simulink model "f6_Central_reservior_demo"  (R2019b)
settings: Solver=VariableStepAuto  StartTime=0.0  StopTime=3  RelTol=1e-3
undefined symbols (not defined in the file): Ion, Lithium
libraries: powerlib x86, powerlib_meascontrol x37, electricdrivelib x1
settings Model: SimulationMode=accelerator  Creator=HALUM  LastModifiedBy=MAHMUD
settings SolverCC: ZeroCrossAlgorithm=Adaptive  AlgebraicLoopSolver=LineSearch
settings DataIOCC: ReturnWorkspaceOutputs=off
settings DebuggingCC: MaskedZcDiagnostic=none  IgnoredZcDiagnostic=none  ArithmeticOperatorsInVariantConditions=warning
settings SFSimCC: SimUseLocalCustomCode=off  CustomCodeUndefinedFunction=UseInterfaceOnly
settings RTWCC: RTWUseLocalCustomCode=off

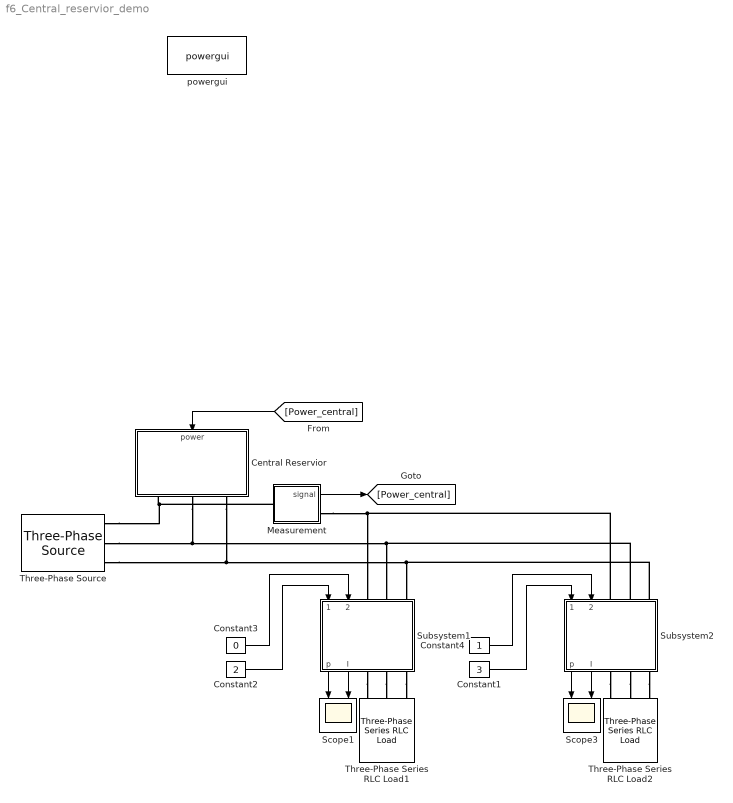
== system f6_Central_reservior_demo ==
  Central Reservior : Subsystem
  Constant1 : Constant  Value=3
  Constant2 : Constant  Value=2
  Constant3 : Constant  Value=0
  Constant4 : Constant
  Measurement : Subsystem
  Scope1 : Scope  NumInputPorts=2
  Scope3 : Scope  NumInputPorts=2
  Subsystem1 : Subsystem
  Subsystem2 : Subsystem
  Three-Phase Series RLC Load1 : powerlib/Elements/Three-Phase Series RLC Load  LConnTagsString=A|B|C  Configuration=Y (grounded)  NominalVoltage=220  Vabc=[1e3 1e3 1e3]  Vabcp=[1e3 1e3 1e3]  NominalFrequency=50  UnbalancedPower=off  ActivePower=200  InductivePower=0  CapacitivePower=0  Pabc=[10e3 9e3 11e3]  QLabc=[100 90 110]  QCabc=[100 90 110]  Pabcp=[10e3 9e3 11e3]  QLabcp=[100 90 110]  QCabcp=[100 90 110]  Measurements=None  LoadType=constant Z
      settings: SourceProductName=Simscape Electrical
  Three-Phase Series RLC Load2 : powerlib/Elements/Three-Phase Series RLC Load  LConnTagsString=A|B|C  Configuration=Y (grounded)  NominalVoltage=220  Vabc=[1e3 1e3 1e3]  Vabcp=[1e3 1e3 1e3]  NominalFrequency=50  UnbalancedPower=off  ActivePower=200  InductivePower=0  CapacitivePower=0  Pabc=[10e3 9e3 11e3]  QLabc=[100 90 110]  QCabc=[100 90 110]  Pabcp=[10e3 9e3 11e3]  QLabcp=[100 90 110]  QCabcp=[100 90 110]  Measurements=None  LoadType=constant Z
      settings: SourceProductName=Simscape Electrical
  Three-Phase Source : powerlib/Electrical Sources/Three-Phase Source  InternalConnection=Yg  VoltagePhases=off  Voltage=1986  PhaseAngle=0  Voltage_phases=[25e3 25e3 25e3]/sqrt(3)  PhaseAngles_phases=[0 -120 +120]  Frequency=50  NonIdealSource=off  SpecifyImpedance=off  Resistance=0.8929  Inductance=0  ShortCircuitLevel=100e6  BaseVoltage=1500  XRratio=7  BusType=swing  Pref=1e3  Qref=0  Prefabc=[10e3, 10e3, 10e3]  Qrefabc=[0, 0, 0]  Qmin=-inf  Qmax=inf
      settings: SourceProductName=Simscape Electrical
  powergui : powerlib/powergui  Priority=1  SimulationMode=Continuous  SampleTime=1e-2  frequency=60  Iterations=50  frequencyindice=50  Pbase=100e6  ErrMax=1e-4  UnitsV=kV  UnitsW=MW  buscounter=0  FunctionMessages=off  echomessages=off  EnableUseOfTLC=off  CurrentSourceSwitches=off  DisableSnubberDevices=off  DisableRonSwitches=off  DisableVfSwitches=off  DisplayEquations=off  AutomaticDiscreteSolvers=off  SolverType=Tustin/Backward Euler (TBE)  Interpol=off  ExternalGateDelay=off  methode=off  Ts=100  x0status=blocks  SPID=on  SwTol=0  HookPort=off  NonlinearTolerance=1e-4  nMaxIteration=100  ContinueOnMaxIteration=off  RestoreLinks=warning  ResistiveCurrentMeasurement=off  Frange=[0:2:500]  Ylog=off  Xlog=on  ShowGrid=off  save=off  variable=ZData  structure=0  ZoomFFT=off  StartTime=0.0  cycles=1  DisplayStyle=1  fundamental=60  FreqAxis=off  MaxFrequency=1000  frequencyindicesteady=1  RmsSteady=1  display=off
      settings: SourceProductName=Simscape Electrical
  wires:
  [Power_central] -> Central Reservior/1(power)
  Subsystem1/1(p) -> Scope1/1
  Subsystem1/2(I) -> Scope1/2
  Constant3/1 -> Subsystem1/2(start time)
  Constant2/1 -> Subsystem1/1(stop time)
  Measurement/1("signal ") -> [Power_central]
  Constant1/1 -> Subsystem2/1(stop time)
  Constant4/1 -> Subsystem2/2(start time)
  Subsystem2/2(I) -> Scope3/2
  Subsystem2/1(p) -> Scope3/1
  connections:
  Subsystem1/RConn3 -- Three-Phase Series RLC Load1/LConn3
  Subsystem1/RConn2 -- Three-Phase Series RLC Load1/LConn2
  Subsystem1/RConn1 -- Three-Phase Series RLC Load1/LConn1
  Central Reservior/RConn3 -- Three-Phase Source/RConn3 -- Subsystem2/LConn3 -- Subsystem1/LConn3
  Central Reservior/RConn2 -- Three-Phase Source/RConn2 -- Subsystem2/LConn2 -- Subsystem1/LConn2
  Measurement/RConn1 -- Subsystem2/LConn1 -- Subsystem1/LConn1
  Measurement/LConn1 -- Three-Phase Source/RConn1 -- Central Reservior/RConn1
  Subsystem2/RConn1 -- Three-Phase Series RLC Load2/LConn1
  Subsystem2/RConn2 -- Three-Phase Series RLC Load2/LConn2
  Subsystem2/RConn3 -- Three-Phase Series RLC Load2/LConn3

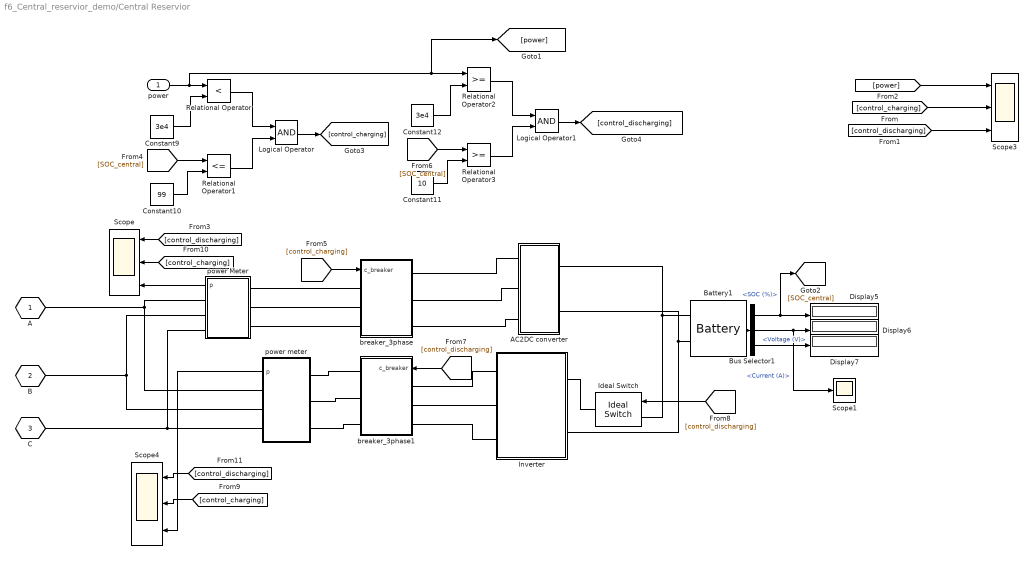
== system f6_Central_reservior_demo/Central Reservior ==
  power : Inport
  AC2DC converter : Subsystem
  Battery1 : electricdrivelib/Extra Sources/Battery  BatType=Lithium-Ion  ShowTempParam=off  ThermalPreset=no  ShowAgeParam=off  NomV=1000  NomQ=1000  SOC=80  Batt_Tr=0.1  PresetModel=on  MaxQ=1000  MinV=750  FullV=1163.9871  Dis_rate=434.7826  R=0.01  Normal_OP=904.3478  expZone="[1080.3859      49.130435]"  current=[6.5 13 32.5]  Units=Time  Tci=20  NomT=20  T2=-30  MaxQ2=4.8  FullV2=7.1  Normal_OP2=5.655  expZone2="[6.58           1]"  Rca=0.6  ti=2000  Dp=0  Neq0=0  Tsim=1e6  Ta1=25  Qeol=5.4*0.9  Reol=0.013333*1.2  Char_age=[2.3478, 3]  Dis_age=[2.3478, 10]  N1=1500  N2=10500  N3=1000  N4=1400  Ta2=45  N5=950
  Bus Selector1 : BusSelector  OutputSignals=SOC (%),Current (A),Voltage (V)
  Constant10 : Constant  Value=99
  Constant11 : Constant  Value=10
  Constant12 : Constant  Value=3e4
  Constant9 : Constant  Value=3e4
  Display5 : Display
  Display6 : Display
  Display7 : Display
  Ideal Switch : powerlib/Power Electronics/Ideal Switch  Ron=0.001  Lon=0  IC=0  Rs=1e5  Cs=inf  Measurements=off
      settings: SourceProductName=Simscape Electrical
  Inverter : Subsystem
  Logical Operator : Logic  AllPortsSameDT=off  OutDataTypeStr=boolean
  Logical Operator1 : Logic  AllPortsSameDT=off  OutDataTypeStr=boolean
  Relational Operator : RelationalOperator  Operator=<  OutDataTypeStr=boolean  ZeroCross=off  RndMeth=Simplest
  Relational Operator1 : RelationalOperator  Operator=<=  OutDataTypeStr=boolean  RndMeth=Simplest
  Relational Operator2 : RelationalOperator  OutDataTypeStr=boolean  ZeroCross=off  RndMeth=Simplest
  Relational Operator3 : RelationalOperator  OutDataTypeStr=boolean  RndMeth=Simplest
  Scope : Scope  NumInputPorts=3
  Scope1 : Scope
  Scope3 : Scope  NumInputPorts=3
  Scope4 : Scope  NumInputPorts=3
  breaker_3phase : Subsystem
  breaker_3phase1 : Subsystem
  power Meter : Subsystem
  power meter : Subsystem
  A : PMIOPort  Tag=PMCPort  Side=Right
  B : PMIOPort  Tag=PMCPort  Port=2  Side=Right
  C : PMIOPort  Tag=PMCPort  Port=3  Side=Right
  wires:
  power/1 -> [power], Relational Operator2/1, Relational Operator/1
  Bus Selector1/2 -> Scope1/1, Display6/1  "<Current (A)>"
  Bus Selector1/3 -> Display7/1  "<Voltage (V)>"
  Battery1/1 -> Bus Selector1/1
  [SOC_central] -> Relational Operator3/1
  Bus Selector1/1 -> [SOC_central], Display5/1  "<SOC (%)>"
  Constant9/1 -> Relational Operator/2
  Logical Operator/1 -> [control_charging]
  Constant10/1 -> Relational Operator1/2
  [SOC_central] -> Relational Operator1/1
  Logical Operator1/1 -> [control_discharging]
  Relational Operator2/1 -> Logical Operator1/1
  Relational Operator1/1 -> Logical Operator/2
  Relational Operator3/1 -> Logical Operator1/2
  Constant11/1 -> Relational Operator3/2
  Constant12/1 -> Relational Operator2/2
  [control_charging] -> breaker_3phase/1(c_breaker)
  [control_discharging] -> Ideal Switch/1
  [control_discharging] -> breaker_3phase1/1(c_breaker)
  Relational Operator/1 -> Logical Operator/1
  [control_discharging] -> Scope3/3
  [control_charging] -> Scope3/2
  [power] -> Scope3/1
  power Meter/1(p) -> Scope/3
  [control_charging] -> Scope/2
  [control_discharging] -> Scope/1
  [control_discharging] -> Scope4/1
  [control_charging] -> Scope4/2
  power meter/1(p) -> Scope4/3
  connections:
  breaker_3phase/RConn3 -- AC2DC converter/LConn3
  Battery1/LConn1 -- Ideal Switch/LConn1 -- AC2DC converter/RConn1
  breaker_3phase/RConn2 -- AC2DC converter/LConn2
  Battery1/LConn2 -- Inverter/LConn2 -- AC2DC converter/RConn2
  breaker_3phase/RConn1 -- AC2DC converter/LConn1
  Ideal Switch/RConn1 -- Inverter/LConn1
  breaker_3phase1/LConn1 -- Inverter/RConn1
  breaker_3phase1/LConn3 -- Inverter/RConn3
  breaker_3phase1/LConn2 -- Inverter/RConn2
  power meter/LConn2 -- breaker_3phase1/RConn2
  power meter/LConn1 -- breaker_3phase1/RConn1
  power meter/LConn3 -- breaker_3phase1/RConn3
  power Meter/LConn3 -- breaker_3phase/LConn3
  power Meter/LConn2 -- breaker_3phase/LConn2
  power Meter/LConn1 -- breaker_3phase/LConn1
  power Meter/RConn1 -- power meter/RConn1 -- A/RConn1
  power Meter/RConn2 -- power meter/RConn2 -- B/RConn1
  power Meter/RConn3 -- power meter/RConn3 -- C/RConn1

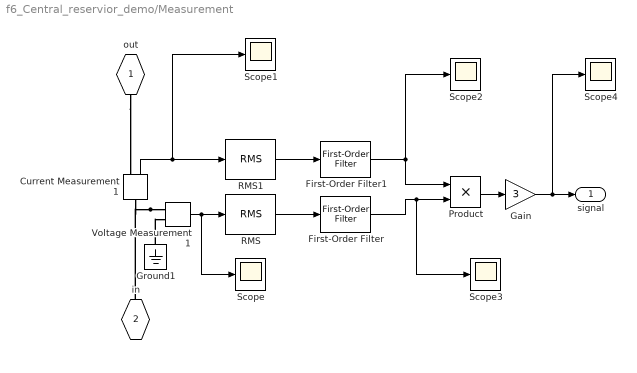
== system f6_Central_reservior_demo/Measurement ==
  Current Measurement1 : powerlib/Measurements/Current Measurement  PhasorSimulation=off  OutputType=Complex  PSBequivalent=0
      settings: SourceProductName=Simscape Electrical
  First-Order Filter : powerlib_meascontrol/Filters/First-Order Filter  FilterType=Lowpass  Tc=100e-3  Ts=0  Initialize=off  Vac_Init=[0, 0, 50]  Vdc_Init=0  PlotResponse=off  FreqRange="[0,  200,  1]"
      settings: SourceProductName=Simscape Electrical
  First-Order Filter1 : powerlib_meascontrol/Filters/First-Order Filter  FilterType=Lowpass  Tc=100e-3  Ts=0  Initialize=off  Vac_Init=[0, 0, 50]  Vdc_Init=0  PlotResponse=off  FreqRange="[0,  200,  1]"
      settings: SourceProductName=Simscape Electrical
  Gain : Gain  Gain=3
  Ground1 : powerlib/Elements/Ground  LConnTagsString=a
      settings: SourceProductName=Simscape Electrical
  Product : Product
  RMS : powerlib_meascontrol/Measurements/RMS  TrueRMS=on  Freq=50  RMSInit=210  Ts=0.001
      settings: SourceProductName=Simscape Electrical
  RMS1 : powerlib_meascontrol/Measurements/RMS  TrueRMS=on  Freq=50  RMSInit=210  Ts=0.001
      settings: SourceProductName=Simscape Electrical
  Scope{,1..4} (5 alike) : Scope
  Voltage Measurement1 : powerlib/Measurements/Voltage Measurement  PhasorSimulation=off  OutputType=Complex  PSBequivalent=0
      settings: SourceProductName=Simscape Electrical
  "out " : PMIOPort  Tag=PMCPort  Side=Right
  in : PMIOPort  Tag=PMCPort  Port=2  Side=Left
  "signal " : Outport
  wires:
  Product/1 -> Gain/1
  First-Order Filter/1 -> Product/2, Scope3/1
  First-Order Filter1/1 -> Scope2/1, Product/1
  Voltage Measurement1/1 -> RMS/1, Scope/1
  RMS1/1 -> First-Order Filter1/1
  RMS/1 -> First-Order Filter/1
  Gain/1 -> Scope4/1, "signal "/1
  Current Measurement1/1 -> RMS1/1, Scope1/1
  connections:
  "out "/RConn1 -- Current Measurement1/RConn1
  Voltage Measurement1/LConn1 -- in/RConn1 -- Current Measurement1/LConn1
  Ground1/LConn1 -- Voltage Measurement1/LConn2

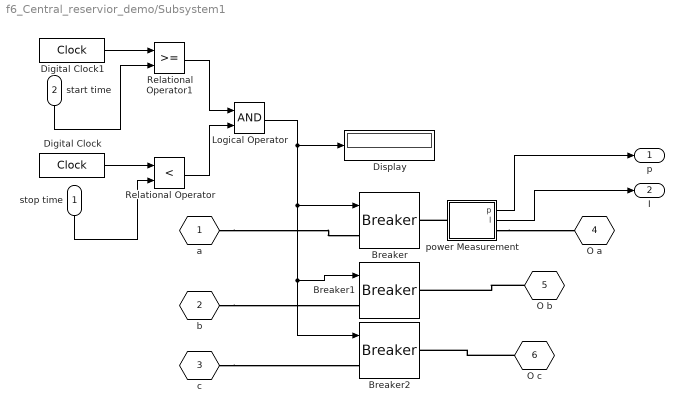
== system f6_Central_reservior_demo/Subsystem1 ==
  stop time : Inport
  start time : Inport  Port=2
  Breaker : powerlib/Elements/Breaker  InitialState=0  SwitchingTimes="[1/60  5/60]"  External=on  BreakerResistance=0.01  SnubberResistance=1e6  SnubberCapacitance=inf  Measurements=None  MoreParameters=on  NoBreakLoop=off
      settings: SourceProductName=Simscape Electrical
  Breaker1 : powerlib/Elements/Breaker  InitialState=0  SwitchingTimes="[1/60  5/60]"  External=on  BreakerResistance=0.01  SnubberResistance=1e6  SnubberCapacitance=inf  Measurements=None  MoreParameters=on  NoBreakLoop=off
      settings: SourceProductName=Simscape Electrical
  Breaker2 : powerlib/Elements/Breaker  InitialState=0  SwitchingTimes="[1/60  5/60]"  External=on  BreakerResistance=0.01  SnubberResistance=1e6  SnubberCapacitance=inf  Measurements=None  MoreParameters=on  NoBreakLoop=off
      settings: SourceProductName=Simscape Electrical
  Digital Clock : DigitalClock
  Digital Clock1 : DigitalClock
  Display : Display
  Logical Operator : Logic  AllPortsSameDT=off  OutDataTypeStr=boolean
  Relational Operator : RelationalOperator  Operator=<  OutDataTypeStr=boolean  RndMeth=Simplest
  Relational Operator1 : RelationalOperator  OutDataTypeStr=boolean  RndMeth=Simplest
  power Measurement : Subsystem
  a : PMIOPort  Tag=PMCPort  Side=Left
  b : PMIOPort  Tag=PMCPort  Port=2  Side=Left
  c : PMIOPort  Tag=PMCPort  Port=3  Side=Left
  "O a " : PMIOPort  Tag=PMCPort  Port=4  Side=Right
  O b : PMIOPort  Tag=PMCPort  Port=5  Side=Right
  O c : PMIOPort  Tag=PMCPort  Port=6  Side=Right
  p : Outport
  I : Outport  Port=2
  wires:
  power Measurement/1(p) -> p/1
  power Measurement/2(I) -> I/1
  Logical Operator/1 -> Breaker/1, Breaker2/1, Breaker1/1, Display/1
  Digital Clock/1 -> Relational Operator/1
  stop time/1 -> Relational Operator/2
  Digital Clock1/1 -> Relational Operator1/1
  start time/1 -> Relational Operator1/2
  Relational Operator1/1 -> Logical Operator/1
  Relational Operator/1 -> Logical Operator/2
  connections:
  power Measurement/LConn1 -- Breaker/RConn1
  power Measurement/RConn1 -- "O a "/RConn1
  O c/RConn1 -- Breaker2/RConn1
  b/RConn1 -- Breaker1/LConn1
  O b/RConn1 -- Breaker1/RConn1
  c/RConn1 -- Breaker2/LConn1
  a/RConn1 -- Breaker/LConn1

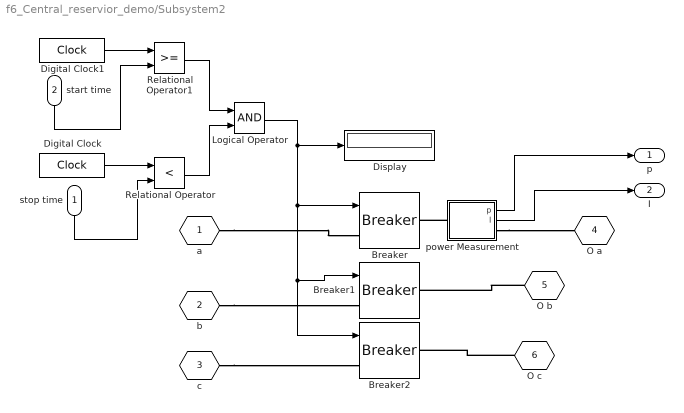
== system f6_Central_reservior_demo/Subsystem2 ==
  stop time : Inport
  start time : Inport  Port=2
  Breaker : powerlib/Elements/Breaker  InitialState=0  SwitchingTimes="[1/60  5/60]"  External=on  BreakerResistance=0.01  SnubberResistance=1e6  SnubberCapacitance=inf  Measurements=None  MoreParameters=on  NoBreakLoop=off
      settings: SourceProductName=Simscape Electrical
  Breaker1 : powerlib/Elements/Breaker  InitialState=0  SwitchingTimes="[1/60  5/60]"  External=on  BreakerResistance=0.01  SnubberResistance=1e6  SnubberCapacitance=inf  Measurements=None  MoreParameters=on  NoBreakLoop=off
      settings: SourceProductName=Simscape Electrical
  Breaker2 : powerlib/Elements/Breaker  InitialState=0  SwitchingTimes="[1/60  5/60]"  External=on  BreakerResistance=0.01  SnubberResistance=1e6  SnubberCapacitance=inf  Measurements=None  MoreParameters=on  NoBreakLoop=off
      settings: SourceProductName=Simscape Electrical
  Digital Clock : DigitalClock
  Digital Clock1 : DigitalClock
  Display : Display
  Logical Operator : Logic  AllPortsSameDT=off  OutDataTypeStr=boolean
  Relational Operator : RelationalOperator  Operator=<  OutDataTypeStr=boolean  RndMeth=Simplest
  Relational Operator1 : RelationalOperator  OutDataTypeStr=boolean  RndMeth=Simplest
  power Measurement : Subsystem
  a : PMIOPort  Tag=PMCPort  Side=Left
  b : PMIOPort  Tag=PMCPort  Port=2  Side=Left
  c : PMIOPort  Tag=PMCPort  Port=3  Side=Left
  "O a " : PMIOPort  Tag=PMCPort  Port=4  Side=Right
  O b : PMIOPort  Tag=PMCPort  Port=5  Side=Right
  O c : PMIOPort  Tag=PMCPort  Port=6  Side=Right
  p : Outport
  I : Outport  Port=2
  wires:
  Relational Operator/1 -> Logical Operator/2
  Relational Operator1/1 -> Logical Operator/1
  start time/1 -> Relational Operator1/2
  Digital Clock1/1 -> Relational Operator1/1
  stop time/1 -> Relational Operator/2
  Digital Clock/1 -> Relational Operator/1
  Logical Operator/1 -> Display/1, Breaker1/1, Breaker2/1, Breaker/1
  power Measurement/2(I) -> I/1
  power Measurement/1(p) -> p/1
  connections:
  a/RConn1 -- Breaker/LConn1
  c/RConn1 -- Breaker2/LConn1
  O b/RConn1 -- Breaker1/RConn1
  b/RConn1 -- Breaker1/LConn1
  O c/RConn1 -- Breaker2/RConn1
  power Measurement/RConn1 -- "O a "/RConn1
  power Measurement/LConn1 -- Breaker/RConn1

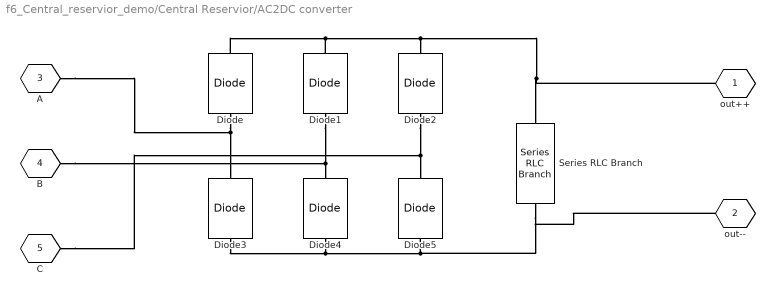
== system f6_Central_reservior_demo/Central Reservior/AC2DC converter ==
  Diode{,1..5} (6 alike) : powerlib/Power Electronics/Diode  Ron=0.001  Lon=0  Vf=0.8  IC=0  UseSnubber=0  Rs=500  Cs=250e-9  Measurements=off
      settings: SourceProductName=Simscape Electrical
  Series RLC Branch : powerlib/Elements/Series RLC Branch  LConnTagsString=__new0  RConnTagsString=__new0  BranchType=C  Resistance=1  Inductance=1e-3  SetiL0=off  InitialCurrent=0  Capacitance=220e-6  Setx0=off  InitialVoltage=0  Measurements=None
      settings: SourceProductName=Simscape Electrical
  out++ : PMIOPort  Tag=PMCPort  Side=Right
  out-- : PMIOPort  Tag=PMCPort  Port=2  Side=Right
  A : PMIOPort  Tag=PMCPort  Port=3  Side=Left
  B : PMIOPort  Tag=PMCPort  Port=4  Side=Left
  C : PMIOPort  Tag=PMCPort  Port=5  Side=Left
  connections:
  Diode/RConn1 -- Diode1/RConn1 -- out++/RConn1 -- Series RLC Branch/RConn1 -- Diode2/RConn1
  Diode3/LConn1 -- Diode4/LConn1 -- out--/RConn1 -- Series RLC Branch/LConn1 -- Diode5/LConn1
  Diode1/LConn1 -- B/RConn1 -- Diode4/RConn1
  Diode/LConn1 -- A/RConn1 -- Diode3/RConn1
  Diode2/LConn1 -- C/RConn1 -- Diode5/RConn1

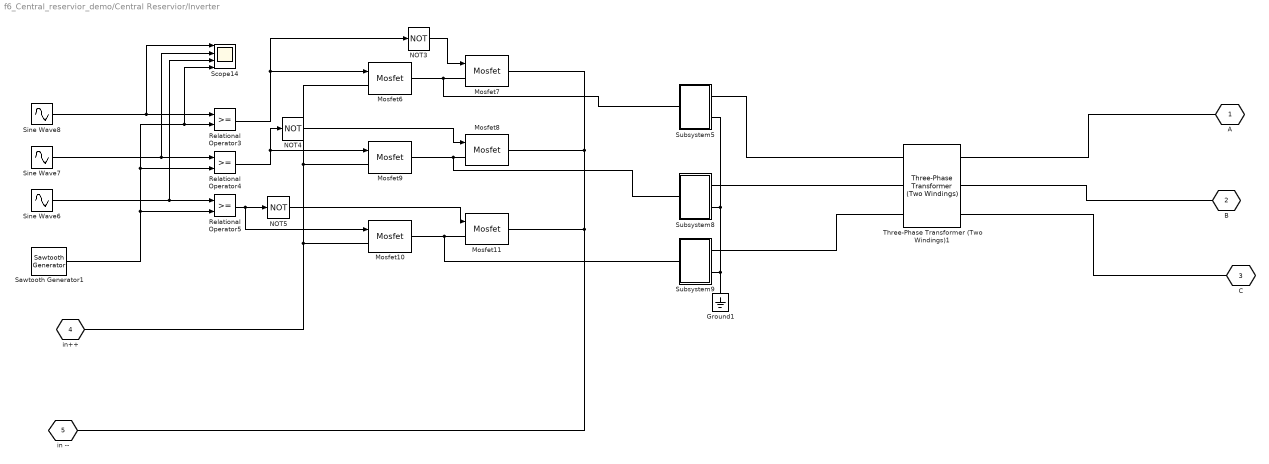
== system f6_Central_reservior_demo/Central Reservior/Inverter ==
  Ground1 : powerlib/Elements/Ground  LConnTagsString=a
      settings: SourceProductName=Simscape Electrical
  Mosfet{6..11} (6 alike) : powerlib/Power Electronics/Mosfet  Ron=0.1  Lon=0  Rd=0.01  Vfd=0  IC=0  Rs=1e5  Cs=inf  Measurements=off
      settings: SourceProductName=Simscape Electrical
  NOT3 : Logic  Operator=NOT  IconShape=distinctive  AllPortsSameDT=off  OutDataTypeStr=boolean
  NOT4 : Logic  Operator=NOT  IconShape=distinctive  AllPortsSameDT=off  OutDataTypeStr=boolean
  NOT5 : Logic  Operator=NOT  IconShape=distinctive  AllPortsSameDT=off  OutDataTypeStr=boolean
  Relational Operator3 : RelationalOperator  OutDataTypeStr=boolean  RndMeth=Simplest
  Relational Operator4 : RelationalOperator  OutDataTypeStr=boolean  RndMeth=Simplest
  Relational Operator5 : RelationalOperator  OutDataTypeStr=boolean  RndMeth=Simplest
  Sawtooth Generator1 : powerlib_meascontrol/Pulse & Signal Generators/Sawtooth Generator  Freq=1e3  Phase=180  Ts=0
      settings: SourceProductName=Simscape Electrical
  Scope14 : Scope  NumInputPorts=4
  Sine Wave6 : Sin  Frequency=2*pi*50  Phase=4*pi/3  SampleTime=0
  Sine Wave7 : Sin  Frequency=2*pi*50  Phase=2*pi/3  SampleTime=0
  Sine Wave8 : Sin  Frequency=2*pi*50  SampleTime=0
  Subsystem5 : Subsystem
  Subsystem8 : Subsystem
  Subsystem9 : Subsystem
  Three-Phase Transformer (Two Windings)1 : powerlib/Elements/Three-Phase Transformer (Two Windings)  Winding1Connection=Yg  Winding2Connection=Yg  CoreType=Three single-phase transformers  SetSaturation=off  Hysteresis=off  DataFile='hysteresis'  SetInitialFlux=off  Measurements=None  UNITS=pu  NominalPower=[ 100e3 , 50 ]  Winding1=[ 338 , 0.002 , 0.08 ]  Winding2=[ 1200 , 0.002 , 0.08 ]  Rm=500  Lm=500  L0=0.5  Saturation=[ 0,0 ; 0.0024,1.2 ; 1.0,1.52 ]  InitialFluxes=[ 0.8 , -0.8 , 0.7 ]  BreakLoop=off  DiscreteSolver=Trapezoidal iterative  DataType=off  TransfoNumber=1
      settings: SourceProductName=Simscape Electrical
  A : PMIOPort  Tag=PMCPort  Side=Right
  B : PMIOPort  Tag=PMCPort  Port=2  Side=Right
  C : PMIOPort  Tag=PMCPort  Port=3  Side=Right
  in++ : PMIOPort  Tag=PMCPort  Port=4  Side=Left
  in -- : PMIOPort  Tag=PMCPort  Port=5  Side=Left
  wires:
  Relational Operator3/1 -> Mosfet6/1, NOT3/1
  Relational Operator5/1 -> NOT5/1, Mosfet10/1
  NOT3/1 -> Mosfet7/1
  Sine Wave8/1 -> Scope14/1, Relational Operator3/1
  Sawtooth Generator1/1 -> Relational Operator5/2, Relational Operator4/2, Scope14/4, Relational Operator3/2
  NOT4/1 -> Mosfet8/1
  Relational Operator4/1 -> NOT4/1, Mosfet9/1
  Sine Wave7/1 -> Scope14/2, Relational Operator4/1
  Sine Wave6/1 -> Scope14/3, Relational Operator5/1
  NOT5/1 -> Mosfet11/1
  connections:
  Subsystem5/RConn2 -- Subsystem8/RConn2 -- Ground1/LConn1 -- Subsystem9/RConn2
  Mosfet11/RConn1 -- in --/RConn1 -- Mosfet8/RConn1 -- Mosfet7/RConn1
  Subsystem5/LConn1 -- Mosfet7/LConn1 -- Mosfet6/RConn1
  Subsystem5/RConn1 -- Three-Phase Transformer (Two Windings)1/LConn1
  Subsystem9/LConn1 -- Mosfet10/RConn1 -- Mosfet11/LConn1
  Three-Phase Transformer (Two Windings)1/LConn2 -- Subsystem8/RConn1
  Subsystem8/LConn1 -- Mosfet8/LConn1 -- Mosfet9/RConn1
  Three-Phase Transformer (Two Windings)1/LConn3 -- Subsystem9/RConn1
  Mosfet6/LConn1 -- Mosfet9/LConn1 -- in++/RConn1 -- Mosfet10/LConn1
  Three-Phase Transformer (Two Windings)1/RConn1 -- A/RConn1
  Three-Phase Transformer (Two Windings)1/RConn2 -- B/RConn1
  Three-Phase Transformer (Two Windings)1/RConn3 -- C/RConn1

== system f6_Central_reservior_demo/Central Reservior/breaker_3phase ==
  c_breaker : Inport
  Breaker : powerlib/Elements/Breaker  InitialState=0  SwitchingTimes="[1/60  5/60]"  External=on  BreakerResistance=0.01  SnubberResistance=1e6  SnubberCapacitance=inf  Measurements=None  MoreParameters=on  NoBreakLoop=off
      settings: SourceProductName=Simscape Electrical
  Breaker1 : powerlib/Elements/Breaker  InitialState=0  SwitchingTimes="[1/60  5/60]"  External=on  BreakerResistance=0.01  SnubberResistance=1e6  SnubberCapacitance=inf  Measurements=None  MoreParameters=on  NoBreakLoop=off
      settings: SourceProductName=Simscape Electrical
  Breaker2 : powerlib/Elements/Breaker  InitialState=0  SwitchingTimes="[1/60  5/60]"  External=on  BreakerResistance=0.01  SnubberResistance=1e6  SnubberCapacitance=inf  Measurements=None  MoreParameters=on  NoBreakLoop=off
      settings: SourceProductName=Simscape Electrical
  a : PMIOPort  Tag=PMCPort  Side=Right
  A : PMIOPort  Tag=PMCPort  Port=2  Side=Left
  B : PMIOPort  Tag=PMCPort  Port=3  Side=Left
  C : PMIOPort  Tag=PMCPort  Port=4  Side=Left
  b : PMIOPort  Tag=PMCPort  Port=5  Side=Right
  c : PMIOPort  Tag=PMCPort  Port=6  Side=Right
  wires:
  c_breaker/1 -> Breaker2/1, Breaker1/1, Breaker/1
  connections:
  C/RConn1 -- Breaker2/LConn1
  b/RConn1 -- Breaker1/RConn1
  a/RConn1 -- Breaker/RConn1
  c/RConn1 -- Breaker2/RConn1
  A/RConn1 -- Breaker/LConn1
  B/RConn1 -- Breaker1/LConn1

== system f6_Central_reservior_demo/Central Reservior/breaker_3phase1 ==
  c_breaker : Inport
  Breaker : powerlib/Elements/Breaker  InitialState=0  SwitchingTimes="[1/60  5/60]"  External=on  BreakerResistance=0.01  SnubberResistance=1e6  SnubberCapacitance=inf  Measurements=None  MoreParameters=on  NoBreakLoop=off
      settings: SourceProductName=Simscape Electrical
  Breaker1 : powerlib/Elements/Breaker  InitialState=0  SwitchingTimes="[1/60  5/60]"  External=on  BreakerResistance=0.01  SnubberResistance=1e6  SnubberCapacitance=inf  Measurements=None  MoreParameters=on  NoBreakLoop=off
      settings: SourceProductName=Simscape Electrical
  Breaker2 : powerlib/Elements/Breaker  InitialState=0  SwitchingTimes="[1/60  5/60]"  External=on  BreakerResistance=0.01  SnubberResistance=1e6  SnubberCapacitance=inf  Measurements=None  MoreParameters=on  NoBreakLoop=off
      settings: SourceProductName=Simscape Electrical
  a : PMIOPort  Tag=PMCPort  Side=Right
  A : PMIOPort  Tag=PMCPort  Port=2  Side=Left
  B : PMIOPort  Tag=PMCPort  Port=3  Side=Left
  C : PMIOPort  Tag=PMCPort  Port=4  Side=Left
  b : PMIOPort  Tag=PMCPort  Port=5  Side=Right
  c : PMIOPort  Tag=PMCPort  Port=6  Side=Right
  wires:
  c_breaker/1 -> Breaker/1, Breaker1/1, Breaker2/1
  connections:
  B/RConn1 -- Breaker1/LConn1
  A/RConn1 -- Breaker/LConn1
  c/RConn1 -- Breaker2/RConn1
  a/RConn1 -- Breaker/RConn1
  b/RConn1 -- Breaker1/RConn1
  C/RConn1 -- Breaker2/LConn1

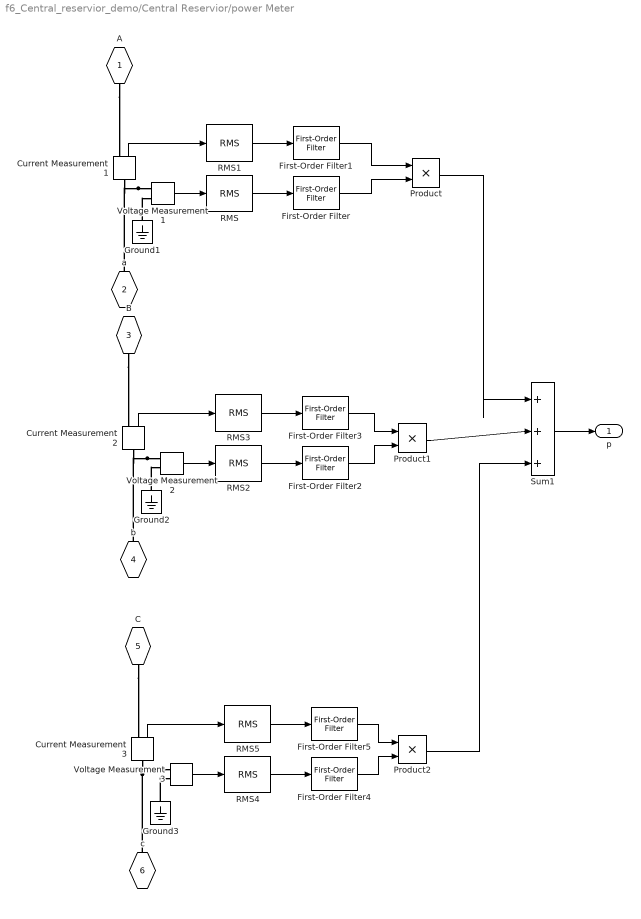
== system f6_Central_reservior_demo/Central Reservior/power Meter ==
  Current Measurement1 : powerlib/Measurements/Current Measurement  PhasorSimulation=off  OutputType=Complex  PSBequivalent=0
      settings: SourceProductName=Simscape Electrical
  Current Measurement2 : powerlib/Measurements/Current Measurement  PhasorSimulation=off  OutputType=Complex  PSBequivalent=0
      settings: SourceProductName=Simscape Electrical
  Current Measurement3 : powerlib/Measurements/Current Measurement  PhasorSimulation=off  OutputType=Complex  PSBequivalent=0
      settings: SourceProductName=Simscape Electrical
  First-Order Filter{,1..5} (6 alike) : powerlib_meascontrol/Filters/First-Order Filter  FilterType=Lowpass  Tc=100e-3  Ts=0  Initialize=off  Vac_Init=[0, 0, 50]  Vdc_Init=0  PlotResponse=off  FreqRange="[0,  200,  1]"
      settings: SourceProductName=Simscape Electrical
  Ground1 : powerlib/Elements/Ground  LConnTagsString=a
      settings: SourceProductName=Simscape Electrical
  Ground2 : powerlib/Elements/Ground  LConnTagsString=a
      settings: SourceProductName=Simscape Electrical
  Ground3 : powerlib/Elements/Ground  LConnTagsString=a
      settings: SourceProductName=Simscape Electrical
  Product : Product
  Product1 : Product
  Product2 : Product
  RMS{,1..5} (6 alike) : powerlib_meascontrol/Measurements/RMS  TrueRMS=on  Freq=50  RMSInit=210  Ts=0.001
      settings: SourceProductName=Simscape Electrical
  Sum1 : Sum  Inputs=|+++
  Voltage Measurement1 : powerlib/Measurements/Voltage Measurement  PhasorSimulation=off  OutputType=Complex  PSBequivalent=0
      settings: SourceProductName=Simscape Electrical
  Voltage Measurement2 : powerlib/Measurements/Voltage Measurement  PhasorSimulation=off  OutputType=Complex  PSBequivalent=0
      settings: SourceProductName=Simscape Electrical
  Voltage Measurement3 : powerlib/Measurements/Voltage Measurement  PhasorSimulation=off  OutputType=Complex  PSBequivalent=0
      settings: SourceProductName=Simscape Electrical
  "A " : PMIOPort  Tag=PMCPort  Side=Right
  a : PMIOPort  Tag=PMCPort  Port=2  Side=Left
  B : PMIOPort  Tag=PMCPort  Port=3  Side=Right
  b : PMIOPort  Tag=PMCPort  Port=4  Side=Left
  C : PMIOPort  Tag=PMCPort  Port=5  Side=Right
  c : PMIOPort  Tag=PMCPort  Port=6  Side=Left
  p : Outport
  wires:
  Product2/1 -> Sum1/3
  Product1/1 -> Sum1/2
  First-Order Filter4/1 -> Product2/2
  First-Order Filter5/1 -> Product2/1
  First-Order Filter2/1 -> Product1/2
  First-Order Filter3/1 -> Product1/1
  Voltage Measurement3/1 -> RMS4/1
  RMS5/1 -> First-Order Filter5/1
  RMS4/1 -> First-Order Filter4/1
  Current Measurement3/1 -> RMS5/1
  Current Measurement2/1 -> RMS3/1
  RMS2/1 -> First-Order Filter2/1
  RMS3/1 -> First-Order Filter3/1
  Voltage Measurement2/1 -> RMS2/1
  Product/1 -> Sum1/1
  First-Order Filter/1 -> Product/2
  First-Order Filter1/1 -> Product/1
  Voltage Measurement1/1 -> RMS/1
  RMS1/1 -> First-Order Filter1/1
  RMS/1 -> First-Order Filter/1
  Sum1/1 -> p/1
  Current Measurement1/1 -> RMS1/1
  connections:
  C/RConn1 -- Current Measurement3/RConn1
  Ground3/LConn1 -- Voltage Measurement3/LConn2
  Current Measurement3/LConn1 -- Voltage Measurement3/LConn1 -- c/RConn1
  Ground2/LConn1 -- Voltage Measurement2/LConn2
  B/RConn1 -- Current Measurement2/RConn1
  Voltage Measurement2/LConn1 -- Current Measurement2/LConn1 -- b/RConn1
  "A "/RConn1 -- Current Measurement1/RConn1
  Voltage Measurement1/LConn1 -- a/RConn1 -- Current Measurement1/LConn1
  Ground1/LConn1 -- Voltage Measurement1/LConn2

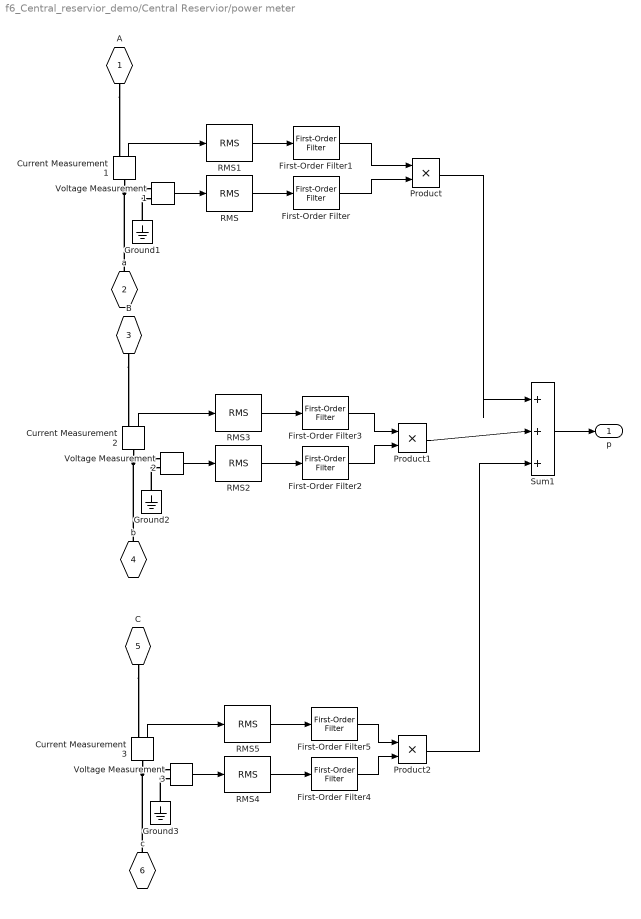
== system f6_Central_reservior_demo/Central Reservior/power meter ==
  Current Measurement1 : powerlib/Measurements/Current Measurement  PhasorSimulation=off  OutputType=Complex  PSBequivalent=0
      settings: SourceProductName=Simscape Electrical
  Current Measurement2 : powerlib/Measurements/Current Measurement  PhasorSimulation=off  OutputType=Complex  PSBequivalent=0
      settings: SourceProductName=Simscape Electrical
  Current Measurement3 : powerlib/Measurements/Current Measurement  PhasorSimulation=off  OutputType=Complex  PSBequivalent=0
      settings: SourceProductName=Simscape Electrical
  First-Order Filter{,1..5} (6 alike) : powerlib_meascontrol/Filters/First-Order Filter  FilterType=Lowpass  Tc=100e-3  Ts=0  Initialize=off  Vac_Init=[0, 0, 50]  Vdc_Init=0  PlotResponse=off  FreqRange="[0,  200,  1]"
      settings: SourceProductName=Simscape Electrical
  Ground1 : powerlib/Elements/Ground  LConnTagsString=a
      settings: SourceProductName=Simscape Electrical
  Ground2 : powerlib/Elements/Ground  LConnTagsString=a
      settings: SourceProductName=Simscape Electrical
  Ground3 : powerlib/Elements/Ground  LConnTagsString=a
      settings: SourceProductName=Simscape Electrical
  Product : Product
  Product1 : Product
  Product2 : Product
  RMS{,1..5} (6 alike) : powerlib_meascontrol/Measurements/RMS  TrueRMS=on  Freq=50  RMSInit=210  Ts=0.001
      settings: SourceProductName=Simscape Electrical
  Sum1 : Sum  Inputs=|+++
  Voltage Measurement1 : powerlib/Measurements/Voltage Measurement  PhasorSimulation=off  OutputType=Complex  PSBequivalent=0
      settings: SourceProductName=Simscape Electrical
  Voltage Measurement2 : powerlib/Measurements/Voltage Measurement  PhasorSimulation=off  OutputType=Complex  PSBequivalent=0
      settings: SourceProductName=Simscape Electrical
  Voltage Measurement3 : powerlib/Measurements/Voltage Measurement  PhasorSimulation=off  OutputType=Complex  PSBequivalent=0
      settings: SourceProductName=Simscape Electrical
  "A " : PMIOPort  Tag=PMCPort  Side=Right
  a : PMIOPort  Tag=PMCPort  Port=2  Side=Left
  B : PMIOPort  Tag=PMCPort  Port=3  Side=Right
  b : PMIOPort  Tag=PMCPort  Port=4  Side=Left
  C : PMIOPort  Tag=PMCPort  Port=5  Side=Right
  c : PMIOPort  Tag=PMCPort  Port=6  Side=Left
  p : Outport
  wires:
  Current Measurement1/1 -> RMS1/1
  Sum1/1 -> p/1
  RMS/1 -> First-Order Filter/1
  RMS1/1 -> First-Order Filter1/1
  Voltage Measurement1/1 -> RMS/1
  First-Order Filter1/1 -> Product/1
  First-Order Filter/1 -> Product/2
  Product/1 -> Sum1/1
  Voltage Measurement2/1 -> RMS2/1
  RMS3/1 -> First-Order Filter3/1
  RMS2/1 -> First-Order Filter2/1
  Current Measurement2/1 -> RMS3/1
  Current Measurement3/1 -> RMS5/1
  RMS4/1 -> First-Order Filter4/1
  RMS5/1 -> First-Order Filter5/1
  Voltage Measurement3/1 -> RMS4/1
  First-Order Filter3/1 -> Product1/1
  First-Order Filter2/1 -> Product1/2
  First-Order Filter5/1 -> Product2/1
  First-Order Filter4/1 -> Product2/2
  Product1/1 -> Sum1/2
  Product2/1 -> Sum1/3
  connections:
  Ground1/LConn1 -- Voltage Measurement1/LConn2
  Current Measurement1/LConn1 -- a/RConn1 -- Voltage Measurement1/LConn1
  "A "/RConn1 -- Current Measurement1/RConn1
  b/RConn1 -- Current Measurement2/LConn1 -- Voltage Measurement2/LConn1
  B/RConn1 -- Current Measurement2/RConn1
  Ground2/LConn1 -- Voltage Measurement2/LConn2
  c/RConn1 -- Voltage Measurement3/LConn1 -- Current Measurement3/LConn1
  Ground3/LConn1 -- Voltage Measurement3/LConn2
  C/RConn1 -- Current Measurement3/RConn1

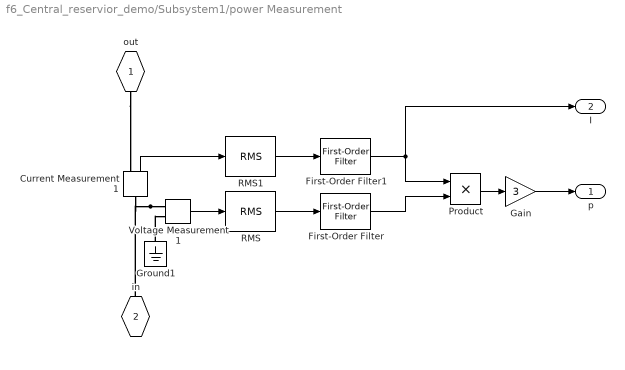
== system f6_Central_reservior_demo/Subsystem1/power Measurement ==
  Current Measurement1 : powerlib/Measurements/Current Measurement  PhasorSimulation=off  OutputType=Complex  PSBequivalent=0
      settings: SourceProductName=Simscape Electrical
  First-Order Filter : powerlib_meascontrol/Filters/First-Order Filter  FilterType=Lowpass  Tc=100e-3  Ts=0  Initialize=off  Vac_Init=[0, 0, 50]  Vdc_Init=0  PlotResponse=off  FreqRange="[0,  200,  1]"
      settings: SourceProductName=Simscape Electrical
  First-Order Filter1 : powerlib_meascontrol/Filters/First-Order Filter  FilterType=Lowpass  Tc=100e-3  Ts=0  Initialize=off  Vac_Init=[0, 0, 50]  Vdc_Init=0  PlotResponse=off  FreqRange="[0,  200,  1]"
      settings: SourceProductName=Simscape Electrical
  Gain : Gain  Gain=3
  Ground1 : powerlib/Elements/Ground  LConnTagsString=a
      settings: SourceProductName=Simscape Electrical
  Product : Product
  RMS : powerlib_meascontrol/Measurements/RMS  TrueRMS=on  Freq=50  RMSInit=210  Ts=0.001
      settings: SourceProductName=Simscape Electrical
  RMS1 : powerlib_meascontrol/Measurements/RMS  TrueRMS=on  Freq=50  RMSInit=210  Ts=0.001
      settings: SourceProductName=Simscape Electrical
  Voltage Measurement1 : powerlib/Measurements/Voltage Measurement  PhasorSimulation=off  OutputType=Complex  PSBequivalent=0
      settings: SourceProductName=Simscape Electrical
  "out " : PMIOPort  Tag=PMCPort  Side=Right
  in : PMIOPort  Tag=PMCPort  Port=2  Side=Left
  p : Outport
  I : Outport  Port=2
  wires:
  Product/1 -> Gain/1
  First-Order Filter/1 -> Product/2
  First-Order Filter1/1 -> Product/1, I/1
  Voltage Measurement1/1 -> RMS/1
  RMS1/1 -> First-Order Filter1/1
  RMS/1 -> First-Order Filter/1
  Gain/1 -> p/1
  Current Measurement1/1 -> RMS1/1
  connections:
  "out "/RConn1 -- Current Measurement1/RConn1
  Voltage Measurement1/LConn1 -- in/RConn1 -- Current Measurement1/LConn1
  Ground1/LConn1 -- Voltage Measurement1/LConn2

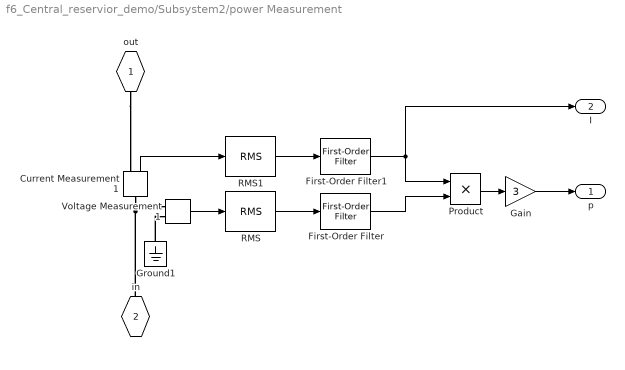
== system f6_Central_reservior_demo/Subsystem2/power Measurement ==
  Current Measurement1 : powerlib/Measurements/Current Measurement  PhasorSimulation=off  OutputType=Complex  PSBequivalent=0
      settings: SourceProductName=Simscape Electrical
  First-Order Filter : powerlib_meascontrol/Filters/First-Order Filter  FilterType=Lowpass  Tc=100e-3  Ts=0  Initialize=off  Vac_Init=[0, 0, 50]  Vdc_Init=0  PlotResponse=off  FreqRange="[0,  200,  1]"
      settings: SourceProductName=Simscape Electrical
  First-Order Filter1 : powerlib_meascontrol/Filters/First-Order Filter  FilterType=Lowpass  Tc=100e-3  Ts=0  Initialize=off  Vac_Init=[0, 0, 50]  Vdc_Init=0  PlotResponse=off  FreqRange="[0,  200,  1]"
      settings: SourceProductName=Simscape Electrical
  Gain : Gain  Gain=3
  Ground1 : powerlib/Elements/Ground  LConnTagsString=a
      settings: SourceProductName=Simscape Electrical
  Product : Product
  RMS : powerlib_meascontrol/Measurements/RMS  TrueRMS=on  Freq=50  RMSInit=210  Ts=0.001
      settings: SourceProductName=Simscape Electrical
  RMS1 : powerlib_meascontrol/Measurements/RMS  TrueRMS=on  Freq=50  RMSInit=210  Ts=0.001
      settings: SourceProductName=Simscape Electrical
  Voltage Measurement1 : powerlib/Measurements/Voltage Measurement  PhasorSimulation=off  OutputType=Complex  PSBequivalent=0
      settings: SourceProductName=Simscape Electrical
  "out " : PMIOPort  Tag=PMCPort  Side=Right
  in : PMIOPort  Tag=PMCPort  Port=2  Side=Left
  p : Outport
  I : Outport  Port=2
  wires:
  Current Measurement1/1 -> RMS1/1
  Gain/1 -> p/1
  RMS/1 -> First-Order Filter/1
  RMS1/1 -> First-Order Filter1/1
  Voltage Measurement1/1 -> RMS/1
  First-Order Filter1/1 -> I/1, Product/1
  First-Order Filter/1 -> Product/2
  Product/1 -> Gain/1
  connections:
  Ground1/LConn1 -- Voltage Measurement1/LConn2
  Current Measurement1/LConn1 -- in/RConn1 -- Voltage Measurement1/LConn1
  "out "/RConn1 -- Current Measurement1/RConn1

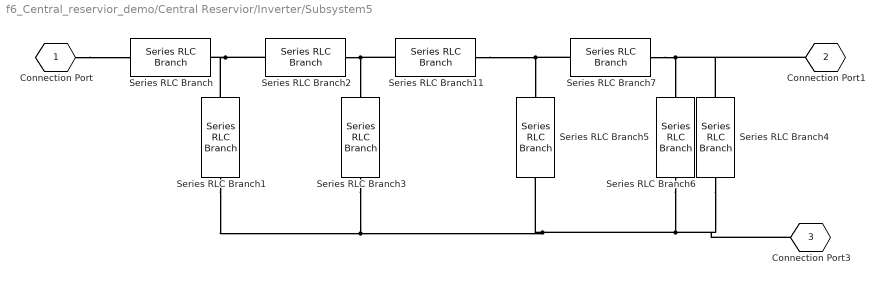
== system f6_Central_reservior_demo/Central Reservior/Inverter/Subsystem5 ==
  Series RLC Branch{,2,5..6} (4 alike) : powerlib/Elements/Series RLC Branch  LConnTagsString=__new0  RConnTagsString=__new0  BranchType=L  Resistance=1  Inductance=92e-3  SetiL0=off  InitialCurrent=0  Capacitance=1e-6  Setx0=off  InitialVoltage=0  Measurements=None
      settings: SourceProductName=Simscape Electrical
  Series RLC Branch1 : powerlib/Elements/Series RLC Branch  LConnTagsString=__new0  RConnTagsString=__new0  BranchType=C  Resistance=1  Inductance=1e-3  SetiL0=off  InitialCurrent=0  Capacitance=110e-6  Setx0=off  InitialVoltage=0  Measurements=None
      settings: SourceProductName=Simscape Electrical
  Series RLC Branch11 : powerlib/Elements/Series RLC Branch  LConnTagsString=__new0  RConnTagsString=__new0  BranchType=R  Resistance=1  Inductance=1e-3  SetiL0=off  InitialCurrent=0  Capacitance=110e-6  Setx0=off  InitialVoltage=0  Measurements=None
      settings: SourceProductName=Simscape Electrical
  Series RLC Branch3 : powerlib/Elements/Series RLC Branch  LConnTagsString=__new0  RConnTagsString=__new0  BranchType=R  Resistance=500  Inductance=1e-3  SetiL0=off  InitialCurrent=0  Capacitance=110e-6  Setx0=off  InitialVoltage=0  Measurements=None
      settings: SourceProductName=Simscape Electrical
  Series RLC Branch4 : powerlib/Elements/Series RLC Branch  LConnTagsString=__new0  RConnTagsString=__new0  BranchType=R  Resistance=10  Inductance=1e-3  SetiL0=off  InitialCurrent=0  Capacitance=110e-6  Setx0=off  InitialVoltage=0  Measurements=None
      settings: SourceProductName=Simscape Electrical
  Series RLC Branch7 : powerlib/Elements/Series RLC Branch  LConnTagsString=__new0  RConnTagsString=__new0  BranchType=C  Resistance=1  Inductance=1e-3  SetiL0=off  InitialCurrent=0  Capacitance=110e-6  Setx0=off  InitialVoltage=0  Measurements=None
      settings: SourceProductName=Simscape Electrical
  Connection Port : PMIOPort  Tag=PMCPort  Side=Left
  Connection Port1 : PMIOPort  Tag=PMCPort  Port=2  Side=Right
  Connection Port3 : PMIOPort  Tag=PMCPort  Port=3  Side=Right
  connections:
  Series RLC Branch7/RConn1 -- Connection Port1/RConn1 -- Series RLC Branch4/RConn1 -- Series RLC Branch6/LConn1
  Series RLC Branch2/RConn1 -- Series RLC Branch11/LConn1 -- Series RLC Branch3/RConn1
  Series RLC Branch1/LConn1 -- Series RLC Branch3/LConn1 -- Connection Port3/RConn1 -- Series RLC Branch4/LConn1 -- Series RLC Branch6/RConn1 -- Series RLC Branch5/RConn1
  Series RLC Branch7/LConn1 -- Series RLC Branch11/RConn1 -- Series RLC Branch5/LConn1
  Series RLC Branch1/RConn1 -- Series RLC Branch2/LConn1 -- Series RLC Branch/RConn1
  Connection Port/RConn1 -- Series RLC Branch/LConn1

== system f6_Central_reservior_demo/Central Reservior/Inverter/Subsystem8 ==
  Series RLC Branch{,2,5..6} (4 alike) : powerlib/Elements/Series RLC Branch  LConnTagsString=__new0  RConnTagsString=__new0  BranchType=L  Resistance=1  Inductance=92e-3  SetiL0=off  InitialCurrent=0  Capacitance=1e-6  Setx0=off  InitialVoltage=0  Measurements=None
      settings: SourceProductName=Simscape Electrical
  Series RLC Branch1 : powerlib/Elements/Series RLC Branch  LConnTagsString=__new0  RConnTagsString=__new0  BranchType=C  Resistance=1  Inductance=1e-3  SetiL0=off  InitialCurrent=0  Capacitance=110e-6  Setx0=off  InitialVoltage=0  Measurements=None
      settings: SourceProductName=Simscape Electrical
  Series RLC Branch11 : powerlib/Elements/Series RLC Branch  LConnTagsString=__new0  RConnTagsString=__new0  BranchType=R  Resistance=1  Inductance=1e-3  SetiL0=off  InitialCurrent=0  Capacitance=110e-6  Setx0=off  InitialVoltage=0  Measurements=None
      settings: SourceProductName=Simscape Electrical
  Series RLC Branch3 : powerlib/Elements/Series RLC Branch  LConnTagsString=__new0  RConnTagsString=__new0  BranchType=R  Resistance=500  Inductance=1e-3  SetiL0=off  InitialCurrent=0  Capacitance=110e-6  Setx0=off  InitialVoltage=0  Measurements=None
      settings: SourceProductName=Simscape Electrical
  Series RLC Branch4 : powerlib/Elements/Series RLC Branch  LConnTagsString=__new0  RConnTagsString=__new0  BranchType=R  Resistance=10  Inductance=1e-3  SetiL0=off  InitialCurrent=0  Capacitance=110e-6  Setx0=off  InitialVoltage=0  Measurements=None
      settings: SourceProductName=Simscape Electrical
  Series RLC Branch7 : powerlib/Elements/Series RLC Branch  LConnTagsString=__new0  RConnTagsString=__new0  BranchType=C  Resistance=1  Inductance=1e-3  SetiL0=off  InitialCurrent=0  Capacitance=110e-6  Setx0=off  InitialVoltage=0  Measurements=None
      settings: SourceProductName=Simscape Electrical
  Connection Port : PMIOPort  Tag=PMCPort  Side=Left
  Connection Port1 : PMIOPort  Tag=PMCPort  Port=2  Side=Right
  Connection Port3 : PMIOPort  Tag=PMCPort  Port=3  Side=Right
  connections:
  Connection Port/RConn1 -- Series RLC Branch/LConn1
  Series RLC Branch/RConn1 -- Series RLC Branch2/LConn1 -- Series RLC Branch1/RConn1
  Series RLC Branch11/RConn1 -- Series RLC Branch7/LConn1 -- Series RLC Branch5/LConn1
  Connection Port3/RConn1 -- Series RLC Branch4/LConn1 -- Series RLC Branch5/RConn1 -- Series RLC Branch1/LConn1 -- Series RLC Branch3/LConn1 -- Series RLC Branch6/RConn1
  Series RLC Branch11/LConn1 -- Series RLC Branch2/RConn1 -- Series RLC Branch3/RConn1
  Connection Port1/RConn1 -- Series RLC Branch4/RConn1 -- Series RLC Branch6/LConn1 -- Series RLC Branch7/RConn1

== system f6_Central_reservior_demo/Central Reservior/Inverter/Subsystem9 ==
  Series RLC Branch{,2,5..6} (4 alike) : powerlib/Elements/Series RLC Branch  LConnTagsString=__new0  RConnTagsString=__new0  BranchType=L  Resistance=1  Inductance=92e-3  SetiL0=off  InitialCurrent=0  Capacitance=1e-6  Setx0=off  InitialVoltage=0  Measurements=None
      settings: SourceProductName=Simscape Electrical
  Series RLC Branch1 : powerlib/Elements/Series RLC Branch  LConnTagsString=__new0  RConnTagsString=__new0  BranchType=C  Resistance=1  Inductance=1e-3  SetiL0=off  InitialCurrent=0  Capacitance=110e-6  Setx0=off  InitialVoltage=0  Measurements=None
      settings: SourceProductName=Simscape Electrical
  Series RLC Branch11 : powerlib/Elements/Series RLC Branch  LConnTagsString=__new0  RConnTagsString=__new0  BranchType=R  Resistance=1  Inductance=1e-3  SetiL0=off  InitialCurrent=0  Capacitance=110e-6  Setx0=off  InitialVoltage=0  Measurements=None
      settings: SourceProductName=Simscape Electrical
  Series RLC Branch3 : powerlib/Elements/Series RLC Branch  LConnTagsString=__new0  RConnTagsString=__new0  BranchType=R  Resistance=500  Inductance=1e-3  SetiL0=off  InitialCurrent=0  Capacitance=110e-6  Setx0=off  InitialVoltage=0  Measurements=None
      settings: SourceProductName=Simscape Electrical
  Series RLC Branch4 : powerlib/Elements/Series RLC Branch  LConnTagsString=__new0  RConnTagsString=__new0  BranchType=R  Resistance=10  Inductance=1e-3  SetiL0=off  InitialCurrent=0  Capacitance=110e-6  Setx0=off  InitialVoltage=0  Measurements=None
      settings: SourceProductName=Simscape Electrical
  Series RLC Branch7 : powerlib/Elements/Series RLC Branch  LConnTagsString=__new0  RConnTagsString=__new0  BranchType=C  Resistance=1  Inductance=1e-3  SetiL0=off  InitialCurrent=0  Capacitance=110e-6  Setx0=off  InitialVoltage=0  Measurements=None
      settings: SourceProductName=Simscape Electrical
  Connection Port : PMIOPort  Tag=PMCPort  Side=Left
  Connection Port1 : PMIOPort  Tag=PMCPort  Port=2  Side=Right
  Connection Port3 : PMIOPort  Tag=PMCPort  Port=3  Side=Right
  connections:
  Series RLC Branch7/RConn1 -- Series RLC Branch6/LConn1 -- Series RLC Branch4/RConn1 -- Connection Port1/RConn1
  Series RLC Branch3/RConn1 -- Series RLC Branch2/RConn1 -- Series RLC Branch11/LConn1
  Series RLC Branch6/RConn1 -- Series RLC Branch1/LConn1 -- Series RLC Branch3/LConn1 -- Series RLC Branch5/RConn1 -- Series RLC Branch4/LConn1 -- Connection Port3/RConn1
  Series RLC Branch5/LConn1 -- Series RLC Branch7/LConn1 -- Series RLC Branch11/RConn1
  Series RLC Branch1/RConn1 -- Series RLC Branch2/LConn1 -- Series RLC Branch/RConn1
  Connection Port/RConn1 -- Series RLC Branch/LConn1
